simulink model "lab3"  (R2023b)
settings: Solver=ode4  StartTime=0.0  StopTime=100.0  FixedStep=0.01  RelTol=1e-3
settings Model: Creator=insomnia  LastModifiedBy=insomnia

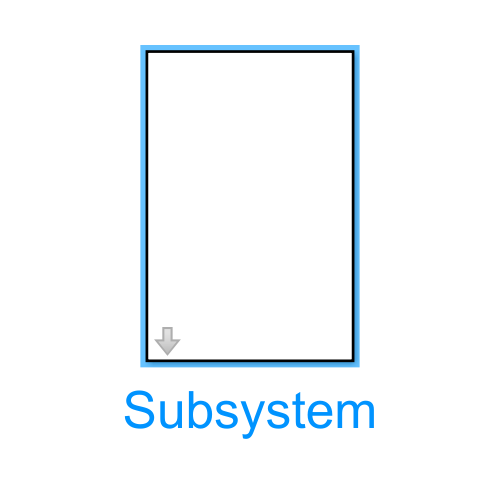
[thumbnail: Simulink's stored preview of the top-level diagram]
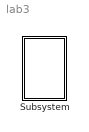
== system lab3 ==
  Subsystem : Subsystem  mask{m=10, k=1, l=3, g=10, fi1=0, fi0=90}
      mask prompts: m "masa"; k "tłumienie"; l "długość liny"; g "grawitacja"; fi1 "prędkość początkowa"; fi0 "kąt początkowy"

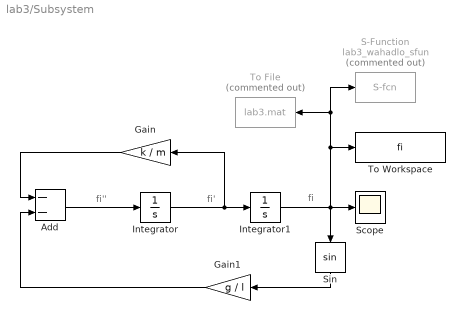
== system lab3/Subsystem ==
  note: fi
  note: fi'
  note: fi''
  Add : Sum  Inputs=--
  Gain : Gain  Gain=k / m
  Gain1 : Gain  Gain=g / l
  Integrator : Integrator  InitialCondition=fi1 * pi / 180
  Integrator1 : Integrator  InitialCondition=fi0 * pi / 180
  S-Function : S-Function  Commented=on  FunctionName=lab3_wahadlo_sfun  Parameters=l, m, fi0  SFunctionDeploymentMode=off  EnableBusSupport=off
  Scope : Scope
  Sin : Trigonometry
  To File : ToFile  Commented=on  Filename=lab3.mat
  To Workspace : ToWorkspace  VariableName=fi  SampleTime=-1
  wires:
  Integrator1/1 -> To Workspace/1, To File/1, S-Function/1, Scope/1, Sin/1
  Integrator/1 -> Gain/1, Integrator1/1
  Gain1/1 -> Add/2
  Add/1 -> Integrator/1
  Gain/1 -> Add/1
  Sin/1 -> Gain1/1
